simulink model "disturbanceEffectOn_first_order_closed"  (R2023b)
settings: Solver=VariableStepAuto  StartTime=0.0  StopTime=10.0  RelTol=1e-3
settings Model: Creator=reemb  LastModifiedBy=reemb

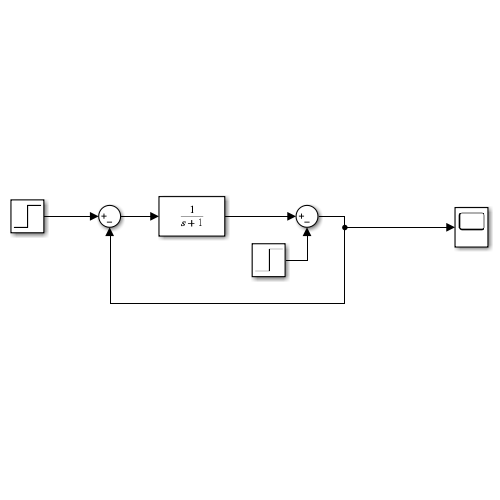
[thumbnail: Simulink's stored preview of the top-level diagram]
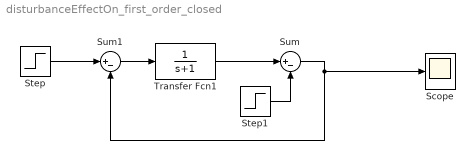
== system disturbanceEffectOn_first_order_closed ==
  Scope : Scope
  Step : Step  SampleTime=0
  Step1 : Step  Time=5  After=0.3  SampleTime=0
  Sum : Sum  Inputs=|+-
  Sum1 : Sum  Inputs=|+-
  Transfer Fcn1 : TransferFcn  Denominator=[1 1]
  wires:
  Sum/1 -> Sum1/2, Scope/1
  Step1/1 -> Sum/2
  Transfer Fcn1/1 -> Sum/1
  Step/1 -> Sum1/1
  Sum1/1 -> Transfer Fcn1/1
